simulink model "simulink_arduino_practice_2019"  (R2018b)
settings: Solver=FixedStepAuto  StartTime=0.0  StopTime=30  RelTol=1e-3  EnableMultiTasking=on
model workspace (MAT data in the model file):
  Threshold = 300
libraries: arduinolib x3
settings Model: ExtModeTrigDuration=2  Creator=gdube  LastModifiedBy=gdube
settings DataIOCC: ReturnWorkspaceOutputs=on
settings OptimizationCC: EnhancedBackFolding=on  PassReuseOutputArgsAs=Individual arguments  ZeroExternalMemoryAtStartup=off  ZeroInternalMemoryAtStartup=off  MaxStackSize=64  OptimizeBlockOrder=speed  DifferentSizesBufferReuse=on  OptimizationCustomize=off
settings DebuggingCC: ParameterTunabilityLossMsg=error
settings HardwareCC: ProdBitPerInt=16  ProdBitPerPointer=16  ProdBitPerSizeT=16  ProdBitPerPtrDiffT=16  ProdLargestAtomicFloat=None  ProdWordSize=8  ProdHWDeviceType=Atmel->AVR
settings SFSimCC: MATLABDynamicMemAlloc=off
settings RTWCC: SystemTargetFile=ert.tlc  HardwareBoard=Arduino Mega 2560  TemplateMakefile=ert_default_tmf  Toolchain=Arduino AVR  BuildConfiguration=Faster Runs
settings CodeAppCC: ForceParamTrailComments=on  IgnoreCustomStorageClasses=off  OperatorAnnotations=on  SimulinkDataObjDesc=on  SFDataObjDesc=on  InsertBlockDesc=on
settings ERTTargetCC: SupportContinuousTime=on  SupportVariableSizeSignals=on  ExtModeStaticAllocSize=2048

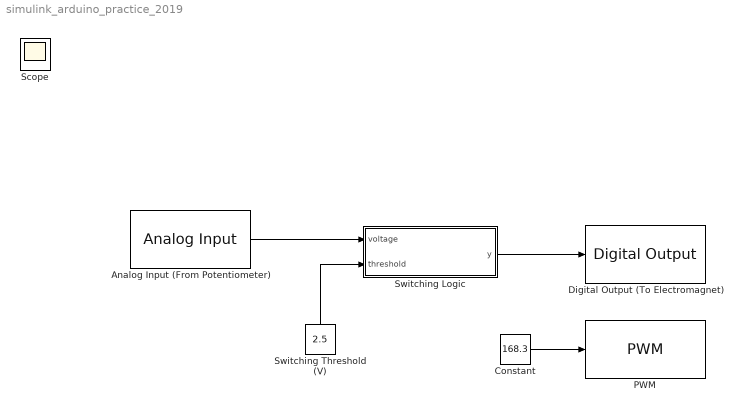
== system simulink_arduino_practice_2019 ==
  Analog Input (From Potentiometer) : arduinolib/Analog Input  pinNumber=0  ReadResultsOnly=off  ConversionTriggerSource=Software  ExternalTriggerType=uint32( 0 )  OutputDataType=uint16  EnableConversionCompleteNotify=off  EnableOuputStatus=off  SampleTime=0.01  blockPlatform=arduino
  Constant : Constant  Value=168.3
  Digital Output (To Electromagnet) : arduinolib/Digital Output  pinNumber=2  Direction=output  blockPlatform=arduino
  PWM : arduinolib/PWM  pinNumber=5  frequencyType=Default  desiredFrequency=490.2  achievableFrequency=490.2
  Switching Logic : MATLAB Function  TreatAsAtomicUnit=on
  Switching Threshold (V) : Constant  Tag=Switching Threshold (V)  Value=2.5
  Scope : Scope
  wires:
  Switching Logic/1(y) -> Digital Output (To Electromagnet)/1
  Switching Threshold (V)/1 -> Switching Logic/2(threshold)
  Analog Input (From Potentiometer)/1 -> Switching Logic/1(voltage)
  Constant/1 -> PWM/1

== matlab function simulink_arduino_practice_2019/Switching Logic ==
  data: voltage input; y output; threshold input
function y = Switch(voltage,threshold)
bins = 1023;
ref_v = 5;
voltage = ref_v/bins * voltage;
if voltage < threshold
            out = 0;
        else
            out = 1;
        end
y = out;
